simulink subsystem "unreal_visualization"  (R2024b)
settings: Solver=VariableStepAuto  StartTime=0.0  StopTime=10.0  RelTol=1e-3
undefined symbols (not defined in the file): att_0, p_0
libraries: sim3dlib x1, uavsim3dlib x1
settings Model: Creator=thesa  LastModifiedBy=thesa
settings RTWCC: GPUComputeCapability=3.5

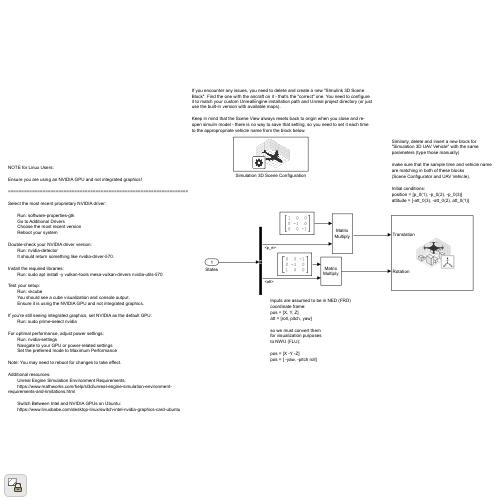
[thumbnail: Simulink's stored preview of the top-level diagram]
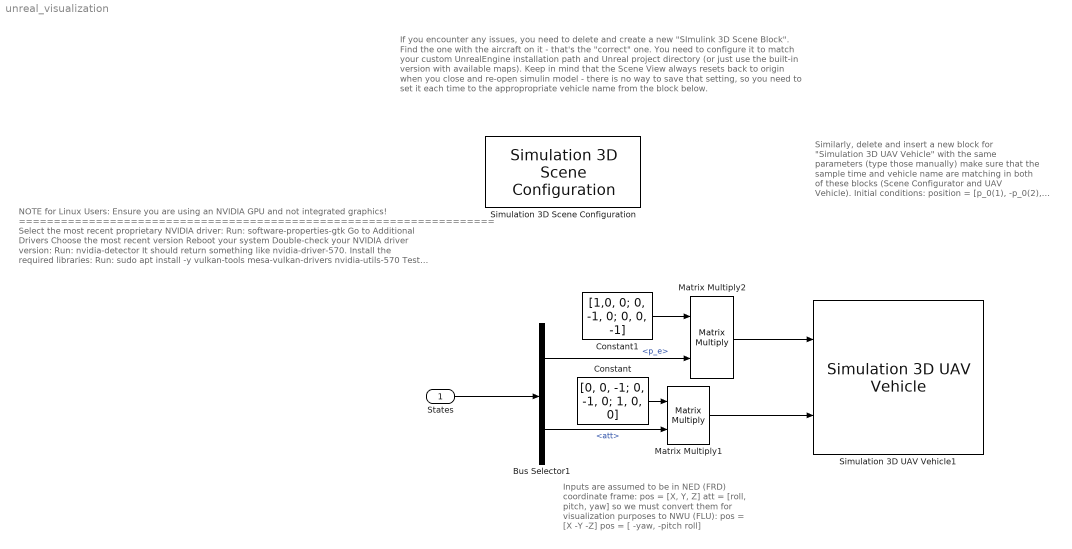
== system unreal_visualization ==
  note: NOTE for Linux Users:
      |
      | Ensure you are using an NVIDIA GPU and not integrated graphics!
      |
      | ====================================================================
      |
      | Select the most recent proprietary NVIDIA driver:
      |
      | 	Run: software-properties-gtk
      | 	Go to Additional Drivers
      | 	Choose the most recent version
      | 	Reboot your system
      |
      | Double-check your NVIDIA driver version:
      | 	Run: nvidia-detector
      | 	It should return something like nvidia-driver-570.
      |
      | Install the required libraries:
      | 	Run: sudo apt install -y vulkan-tools mesa-vulkan-drivers nvidia-utils-570
      |
      | Test your setup:
      | 	Run: vkcube
      | 	You should see a cube visualization and console output.
      | 	Ensure it is using the NVIDIA GPU and not integrated graphics.
      |
      | If you're still seeing integrated graphics, set NVIDIA as the default GPU:
      | 	Run: sudo prime-select nvidia
      |
      | For optimal performance, adjust power settings:
      | 	Run: nvidia-settings
      | 	Navigate to your GPU or power-related settings
      | 	Set the preferred mode to Maximum Performance
      |
      | Note: You may need to reboot for changes to take effect.
      |
      | Additional resources:
      | 	Unreal Engine Simulation Environment Requirements:
      | 	https://www.mathworks.com/help/sl3d/unreal-engine-simulation-environment-requirements-and-limitations.html
      |
      | 	Switch Between Intel and NVIDIA GPUs on Ubuntu:
      | 	https://www.linuxbabe.com/desktop-linux/switch-intel-nvidia-graphics-card-ubuntu
  note: Inputs are assumed to be in NED (FRD)
      | coordinate frame:
      | pos = [X, Y, Z]
      | att = [roll, pitch, yaw]
      |
      | so we must convert them
      | for visualization purposes
      | to NWU (FLU):
      |
      | pos = [X -Y -Z]
      | pos = [ -yaw, -pitch roll]
  note: Similarly, delete and insert a new block for
      | "Simulation 3D UAV Vehicle" with the same
      | parameters (type those manually)
      |
      | make sure that the sample time and vehicle name
      | are matching in both of these blocks
      | (Scene Configurator and UAV Vehicle).
      |
      | Initial conditions:
      | position = [p_0(1), -p_0(2), -p_0(3)]
      | attitude = [-att_0(3), -att_0(2), att_0(1)]
  note: If you encounter any issues, you need to delete and create a new "SImulink 3D Scene Block". Find the one with the aircraft on it - that's the "correct" one. You need to configure it to match your custom UnrealEngine installation path and Unreal project directory (or just use the built-in version with available maps).
      |
      | Keep in mind that the Scene View always resets back to origin when you close and re-open simulin model - there is no way to save that setting, so you need to set it each time
      | to the appropropriate vehicle name from the block below.
  States : Inport
  Bus Selector1 : BusSelector  OutputSignals=p_e,att
  Constant : Constant  Value=[0, 0, -1; 0, -1, 0; 1, 0, 0]
  Constant1 : Constant  Value=[1,0, 0; 0, -1, 0; 0, 0, -1]
  Matrix Multiply1 : Product  Multiplication=Matrix(*)
  Matrix Multiply2 : Product  Multiplication=Matrix(*)
  Simulation 3D Scene Configuration : sim3dlib/Simulation 3D Scene Configuration  Priority=0  ProjectFormat=Default Scenes  SceneDesc=Airport  ProjectName=C:\Program Files\MATLAB\R2024b\toolbox\shared\sim3d_projects\automotive_project_windows\UE\WindowsNoEditor\VehicleSimulation.exe  ScenePath=GriffissAirport  UEProjPath=/home/jack/UnrealEngine/UnrealEngine-5.3.0/Projects/matlab/AutoVrtlEnv/AutoVrtlEnv.uproject  EnableOpenDRIVE=off  vehTagList={'Scene Origin'}  vehTag=Scene Origin  FreeCameraInitialTranslation=[3532+(6550.01-3532)/2, 200, 0.1]  FreeCameraDefaultInitialTranslation=[-6, 0, 2]  FreeCameraInitialRotation=[0, -15, 0]  FreeCameraDefaultInitialRotation=[0, -15, 0]  OpVisEn=off  Ts=1/50  EnableWindow=on  EnableRemoteAccess=off  EnableWeather=off  SunAzimuth=90  SunAltitude=40.0  EnableGeospatialSun=off  Latitude=0  Longitude=0  Date=2023-01-01  Time=10:30:00  GeoTimeZone=-5.0  SunDaylightSaving=off  wind=1  clouds=10  EnableVolumetricClouds=off  CloudCoverage=0  CloudAltitude=6  fog=0  rain=0  RaindropsEffect=off  SnowDensity=0  EnableGeospatial=off  UseTrueOrigin=off  OriginHeight=200  OriginLatitude=40.744652  OriginLongitude=-73.988864  MapStyle=Aerial  AdditionalAssetIDs=[]  UseAdvancedSunSky=off  SolarTime=11  TimeZone=-5  Day=21  Month=9  Year=2022  UseDaylightSavingTime=on  DSTStartDay=10  DSTStartMonth=3  DSTEndDay=3  DSTEndMonth=11  DSTSwitchHour=2  sensorTag=MainCamera1  sensorId=1  sensorName=MainCamera1  mountLoc=Origin  offsetFlag=off  tmountOffset=[0, 0, 0]  rmountOffset=[0, 0, 0]  HorizontalResolution=1280  VerticalResolution=720  HorizontalFOV=60  mountPoint=[0 0 0]  mountOrientation=[0 0 0]  aMode=0  ID=1  GeoTrigger=Inactive
      settings: LibrarySourceBlock=aerolibsim3d/Simulation 3D Scene Configuration
  Simulation 3D UAV Vehicle1 : uavsim3dlib/Simulation 3D UAV Vehicle  Priority=-1  Mesh=Quadrotor  MeshPath=/MathWorksUAVContent/UAVs/HexaRotorUAV/HexaRotor.HexaRotor  Color=Orange  ActorName=SimulinkVehicle1  UseGlobalFrame=off  InitialTranslation=[p_0(1), -p_0(2), -p_0(3)]  InitialRotation=[-att_0(3), -att_0(2), att_0(1)]  InitialTranslationGlobal=[0 0 0]  InitialGeoOrigin=[0 0 0]  InitialRotationGlobal=[0 0 0]  SampleTime=1/50  ActorType=SimulinkVehicle  ID=1  aMode=4  ActorTag=SimulinkVehicle1
  wires:
  Constant1/1 -> Matrix Multiply2/1
  Matrix Multiply1/1 -> Simulation 3D UAV Vehicle1/2
  Bus Selector1/2 -> Matrix Multiply1/2  "<att>"
  Bus Selector1/1 -> Matrix Multiply2/2  "<p_e>"
  Constant/1 -> Matrix Multiply1/1
  Matrix Multiply2/1 -> Simulation 3D UAV Vehicle1/1
  States/1 -> Bus Selector1/1
